simulink model "AEBWithSensorFusionMdlRef"  (R2020b)
settings: Solver=FixedStepAuto  StartTime=0.0  StopTime=34  FixedStep=0.1  RelTol=1e-3
undefined symbols (not defined in the file or in its folder): M, N, numCoasts, posSelector, speedController, Ts, v_set
libraries: drivinglib x2, pid_lib x1
settings Model: Creator=The MathWorks, Inc.  LastModifiedBy=chiar
settings SolverCC: MinimalZcImpactIntegration=on
settings DataIOCC: SaveOutput=off  SignalLogging=off  SaveTime=off  ReturnWorkspaceOutputs=off
settings OptimizationCC: DefaultParameterBehavior=Inlined  InlineInvariantSignals=on  PassReuseOutputArgsAs=Individual arguments  ZeroExternalMemoryAtStartup=off  ZeroInternalMemoryAtStartup=off  OptimizeBlockOrder=speed  EfficientTunableParamExpr=on
settings DebuggingCC: ParameterTunabilityLossMsg=error  ArithmeticOperatorsInVariantConditions=warning
settings HardwareCC: ProdLongLongMode=on
settings ModelReferenceCC: PropagateVarSize=Only when enabling
settings SFSimCC: SimUseLocalCustomCode=off  MATLABDynamicMemAlloc=off  CustomCodeUndefinedFunction=UseInterfaceOnly  SimTargetLang=C++
settings RTWCC: Description=Embedded Coder  SystemTargetFile=ert.tlc  TemplateMakefile=ert_default_tmf  GenerateReport=on  RTWUseLocalCustomCode=off  BuildConfiguration=Faster Runs  IncludeHyperlinkInReport=on  LaunchReport=on  TargetLang=C++  GenerateTraceInfo=on  GenerateTraceReport=on  GenerateTraceReportSl=on  GenerateTraceReportSf=on  GenerateTraceReportEml=on  GenerateCodeMetricsReport=on
settings CodeAppCC: ForceParamTrailComments=on  IgnoreCustomStorageClasses=off  MaxIdLength=63  OperatorAnnotations=on  SimulinkDataObjDesc=on  SFDataObjDesc=on  CustomSymbolStrFcn=$N$M$F  InsertBlockDesc=on
settings ERTTargetCC: TargetLangStandard=C++03 (ISO)  GenerateSampleERTMain=on  CombineSignalStateStructs=on  SuppressErrorStatus=on  CodeInterfacePackaging=C++ class  InlinedParameterPlacement=NonHierarchical  RootIOFormat=Structure reference  RTWCAPISignals=on  ERTCustomFileTemplate=example_file_process.tlc

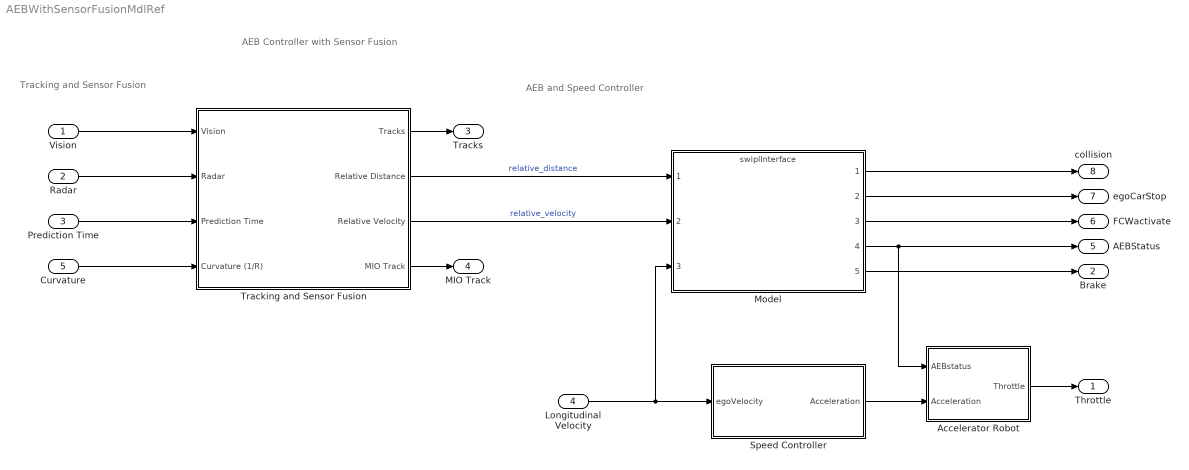
== system AEBWithSensorFusionMdlRef ==
  note: AEB and Speed Controller
  note: Tracking and Sensor Fusion
  note: AEB Controller with Sensor Fusion
  Vision : Inport  OutDataTypeStr=Bus: BusVision  PortDimensions=[1 1]  SampleTime=[0.10000000000000001,0]  BusOutputAsStruct=on
  Radar : Inport  Port=2  OutDataTypeStr=Bus: BusRadar  PortDimensions=[1 1]  SampleTime=[0.10000000000000001,0]  BusOutputAsStruct=on
  Prediction Time : Inport  Port=3  OutDataTypeStr=double  PortDimensions=[1 1]  SampleTime=[0.10000000000000001,0]  BusOutputAsStruct=on
  Longitudinal Velocity : Inport  Port=4  OutDataTypeStr=double  PortDimensions=1  SampleTime=[0.10000000000000001,0]
  Curvature : Inport  Port=5  OutDataTypeStr=double  PortDimensions=[1 1]  SampleTime=[0.10000000000000001,0]  BusOutputAsStruct=on
  Accelerator Robot : Subsystem
  Model : ModelReference  ModelNameDialog=swiplInterface.slx  SimulationMode=Normal  ModelReferenceVersion=1.2
  Speed Controller : Subsystem
  Tracking and Sensor Fusion : Subsystem  TreatAsAtomicUnit=on
      settings: RTWFileNameOpts=Use function name
  "Throttle " : Outport  OutDataTypeStr=double  PortDimensions=1  SampleTime=[0.10000000000000001,0]  VectorParamsAs1DForOutWhenUnconnected=off
  Brake : Outport  Port=2  OutDataTypeStr=double  PortDimensions=1  SampleTime=[0.10000000000000001,0]  VectorParamsAs1DForOutWhenUnconnected=off
  Tracks : Outport  Port=3  OutDataTypeStr=Bus:BusMultiObjectTracker1  PortDimensions=[1 1]  SampleTime=[0.10000000000000001,0]  VectorParamsAs1DForOutWhenUnconnected=off  BusOutputAsStruct=on
  MIO Track : Outport  Port=4  OutDataTypeStr=double  PortDimensions=1  SampleTime=[0.10000000000000001,0]  VectorParamsAs1DForOutWhenUnconnected=off
  AEBStatus : Outport  Port=5  OutDataTypeStr=uint8  PortDimensions=1  SampleTime=[0.10000000000000001,0]  VectorParamsAs1DForOutWhenUnconnected=off
  FCWactivate : Outport  Port=6  OutDataTypeStr=uint8  PortDimensions=1  SampleTime=[0.10000000000000001,0]  VectorParamsAs1DForOutWhenUnconnected=off
  egoCarStop : Outport  Port=7  PortDimensions=1  SampleTime=[0.10000000000000001,0]  VectorParamsAs1DForOutWhenUnconnected=off
  collision : Outport  Port=8  PortDimensions=1  SampleTime=[0.10000000000000001,0]  VectorParamsAs1DForOutWhenUnconnected=off
  wires:
  Tracking and Sensor Fusion/1(Tracks) -> Tracks/1
  Vision/1 -> Tracking and Sensor Fusion/1(Vision)
  Radar/1 -> Tracking and Sensor Fusion/2(Radar)
  Prediction Time/1 -> Tracking and Sensor Fusion/3(Prediction Time)
  Curvature/1 -> Tracking and Sensor Fusion/4(Curvature (1/R))
  Tracking and Sensor Fusion/4(MIO Track) -> MIO Track/1
  Longitudinal Velocity/1 -> Model/3, Speed Controller/1(egoVelocity)
  Tracking and Sensor Fusion/2(Relative Distance) -> Model/1  "relative_distance"
  Model/4 -> Accelerator Robot/1(AEBstatus), AEBStatus/1
  Tracking and Sensor Fusion/3(Relative Velocity) -> Model/2  "relative_velocity"
  Model/2 -> egoCarStop/1
  Model/1 -> collision/1
  Model/3 -> FCWactivate/1
  Model/5 -> Brake/1
  Speed Controller/1(Acceleration) -> Accelerator Robot/2(Acceleration)
  Accelerator Robot/1(Throttle) -> "Throttle "/1

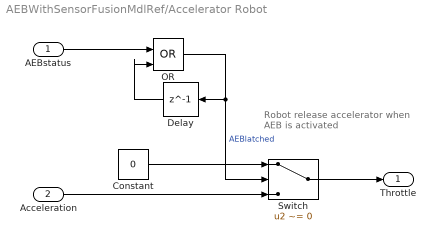
== system AEBWithSensorFusionMdlRef/Accelerator Robot ==
  note: Robot release accelerator when AEB is activated
  AEBstatus : Inport
  Acceleration : Inport  Port=2
  Constant : Constant  Value=0
  Delay : Delay  DelayLength=1
  OR : Logic  Operator=OR  IconShape=distinctive  AllPortsSameDT=off  OutDataTypeStr=boolean
  Switch : Switch  Criteria=u2 ~= 0
  Throttle : Outport  VectorParamsAs1DForOutWhenUnconnected=off
  wires:
  OR/1 -> Delay/1, Switch/2  "AEBlatched"
  Delay/1 -> OR/2
  Switch/1 -> Throttle/1
  AEBstatus/1 -> OR/1
  Constant/1 -> Switch/1
  Acceleration/1 -> Switch/3

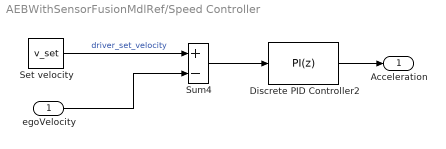
== system AEBWithSensorFusionMdlRef/Speed Controller ==
  egoVelocity : Inport
  Discrete PID Controller2 : pid_lib/PID Controller  Controller=PI  Form=Parallel  TimeDomain=Discrete-time  UseExternalTs=off  SampleTime=-1  IntegratorMethod=Forward Euler  FilterMethod=Forward Euler  ControllerParametersSource=internal  P=speedController.Kp  I=speedController.Ki  D=speedController.Kd  UseFilter=on  N=speedController.FilterCoeff  TunerSelectOption=Transfer Function Based (PID Tuner App)  InitialConditionSource=internal  InitialConditionForIntegrator=0  InitialConditionForFilter=0  DifferentiatorICPrevScaledInput=0  ExternalReset=none  TrackingMode=off  Kt=1  LimitOutput=on  SatLimitsSource=internal  UpperSaturationLimit=speedController.Amax  LowerSaturationLimit=speedController.Amin  LinearizeAsGain=off  AntiWindupMode=clamping  Kb=1  POutMin=[]  POutMax=[]  IOutMin=[]  IOutMax=[]  DOutMin=[]  DOutMax=[]  NOutMin=[]  NOutMax=[]  SumOutMin=[]  SumOutMax=[]  SaturationOutMin=[]  SaturationOutMax=[]  PParamMin=[]  PParamMax=[]  IParamMin=[]  IParamMax=[]  DParamMin=[]  DParamMax=[]  NParamMin=[]  NParamMax=[]  KbParamMin=[]  KbParamMax=[]  KtParamMin=[]  KtParamMax=[]  KbOutMin=[]  KbOutMax=[]  KtOutMin=[]  KtOutMax=[]  IntegratorOutMin=[]  IntegratorOutMax=[]  FilterOutMin=[]  FilterOutMax=[]  SumI1OutMin=[]  SumI1OutMax=[]  SumI2OutMin=[]  SumI2OutMax=[]  SumI3OutMin=[]  SumI3OutMax=[]  SumI4OutMin=[]  SumI4OutMax=[]  SumDOutMin=[]  SumDOutMax=[]  DifferentiatorOutMin=[]  DifferentiatorOutMax=[]  FilterDiffOutCoefMin=[]  FilterDiffOutCoefMax=[]  ReciprocalOutMin=[]  ReciprocalOutMax=[]  SumDenOutMin=[]  SumDenOutMax=[]  SumNumOutMin=[]  SumNumOutMax=[]  DivideOutMin=[]  DivideOutMax=[]  UdiffTsProdOutMin=[]  UdiffTsProdOutMax=[]  NTsProdOutMin=[]  NTsProdOutMax=[]  UintegralTsProdOutMin=[]  UintegralTsProdOutMax=[]  UngainTsProdOutMin=[]  UngainTsProdOutMax=[]  IntegratorContinuousStateAttributes=''  IntegratorStateMustResolveToSignalObject=off  IntegratorRTWStateStorageClass=Auto  FilterContinuousStateAttributes=''  FilterStateMustResolveToSignalObject=off  FilterRTWStateStorageClass=Auto  ParallelPVariant=InternalParameters  IdealPVariant=Disabled  IVariant=InternalParameters  DVariant=Disabled  IntegratorVariant=Discrete  SatVariant=Enabled  AWVariant=DiscClampingParallel  PCopyVariant=Disabled  TRVariant=Disabled  FdbkBlocksVariant=Forward  IdealPFdbkVariant=Disabled  SatFdbkVariant=Disabled  DerivativeFilterVariant=Disabled  NVariant=Disabled  NCopyVariant=Disabled_SignalSpec  FilterICVariant=Disabled  IntegratorICVariant=InternalICs  ExternalResetVariant=Disabled  TRSumVariant=Passthrough  SumFdbkVariant=Disabled  SumVariant=Sum_PI  TsampFilterVariant=InternalTs  TsampNgainVariant=Passthrough  TsampIntegralVariant=Passthrough  ExternalSaturationOutDataTypeStr=Inherit: Same as second input
  Set velocity : Constant  Value=v_set  SampleTime=Ts
  Sum4 : Sum  Inputs=+-
  Acceleration : Outport  VectorParamsAs1DForOutWhenUnconnected=off
  wires:
  Set velocity/1 -> Sum4/1  "driver_set_velocity"
  egoVelocity/1 -> Sum4/2
  Discrete PID Controller2/1 -> Acceleration/1
  Sum4/1 -> Discrete PID Controller2/1

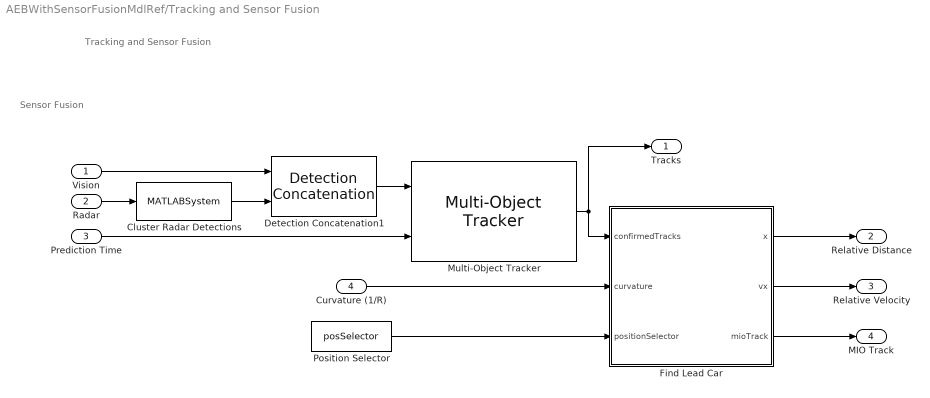
== system AEBWithSensorFusionMdlRef/Tracking and Sensor Fusion ==
  note: Sensor Fusion
  note: Tracking and Sensor Fusion
  Vision : Inport  OutDataTypeStr=Bus: BusVision  PortDimensions=[1 1]  SampleTime=[0.10000000000000001,0]  BusOutputAsStruct=on
  Radar : Inport  Port=2  OutDataTypeStr=Bus: BusRadar  PortDimensions=[1 1]  SampleTime=[0.10000000000000001,0]  BusOutputAsStruct=on
  Prediction Time : Inport  Port=3  OutDataTypeStr=double  PortDimensions=[1 1]  SampleTime=[0.10000000000000001,0]  BusOutputAsStruct=on
  Curvature (1/R) : Inport  Port=4  OutDataTypeStr=double  PortDimensions=[1 1]  SampleTime=[0.10000000000000001,0]  BusOutputAsStruct=on
  Cluster Radar Detections : MATLABSystem  System=helperClusterDetections  ClusterSize=clusterSize  BusNameSource=Auto  BusName=BusClusterDetections  SimulateUsing=Interpreted execution
      mask Type: helperClusterDetections
      mask Display:
      | disp(['Detection' char(10) 'Clustering']);
      | port_label('input',1,'In');
      | port_label('output',1,'Out');
  Detection Concatenation1 : drivinglib/Detection Concatenation  NumInputs=2  BusNameSource=Auto  BusName=BusDetectionConcatenation1  SimulateUsing=Interpreted execution
      settings: SourceProductName=Automated Driving Toolbox
  Find Lead Car : MATLAB Function  TreatAsAtomicUnit=on
  Multi-Object Tracker : drivinglib/Multi-Object Tracker  TrackerIndex=uint32( 0 )  FilterInitializationFcn=initcvekf  AssignmentThreshold=assigThresh  ConfirmationThreshold=[M,N]  DeletionThreshold=[numCoasts,numCoasts]  MaxNumTracks=numTracks  MaxNumSensors=numSensors  StateParams=struct  TimeInputSource=Input port  HasCostMatrixInput=off  HasDetectableTrackIDsInput=off  BusNameSource=Property  BusName=BusMultiObjectTracker1  TentativeTracksOutputPort=off  AllTracksOutputPort=off  SimulateUsing=Interpreted execution
      settings: SourceProductName=Automated Driving Toolbox
  Position Selector : Constant  Value=posSelector
  Tracks : Outport  OutDataTypeStr=Bus:BusMultiObjectTracker1  PortDimensions=[1 1]  SampleTime=[0.10000000000000001,0]  VectorParamsAs1DForOutWhenUnconnected=off  BusOutputAsStruct=on
  Relative Distance : Outport  Port=2  VectorParamsAs1DForOutWhenUnconnected=off
  Relative Velocity : Outport  Port=3  VectorParamsAs1DForOutWhenUnconnected=off
  MIO Track : Outport  Port=4  VectorParamsAs1DForOutWhenUnconnected=off
  wires:
  Find Lead Car/3(mioTrack) -> MIO Track/1
  Cluster Radar Detections/1 -> Detection Concatenation1/2
  Vision/1 -> Detection Concatenation1/1
  Prediction Time/1 -> Multi-Object Tracker/2
  Find Lead Car/2(vx) -> Relative Velocity/1
  Radar/1 -> Cluster Radar Detections/1
  Curvature (1/R)/1 -> Find Lead Car/2(curvature)
  Multi-Object Tracker/1 -> Find Lead Car/1(confirmedTracks), Tracks/1
  Detection Concatenation1/1 -> Multi-Object Tracker/1
  Find Lead Car/1(x) -> Relative Distance/1
  Position Selector/1 -> Find Lead Car/3(positionSelector)

== matlab function AEBWithSensorFusionMdlRef/Tracking and Sensor Fusion/Find Lead Car ==
  data: confirmedTracks input; x output double size=[1 1]; vx output size=[1 1]; curvature input; mioTrack output; positionSelector input
function [x,vx,mioTrack] = findLeadCar(confirmedTracks, curvature, positionSelector)
% This function finds the lead car: a car in front of the ego car that
% satisfies all the criteria below:
% * Within the ego car's lane.
% * In front of the ego car.
% * Closest to the ego car.

% Important notes:
% 1. If you change state definition, change the following:
%       State = [x;vx;y;vy;z;vz] (3D constant velocity)
numStates = 6;

% 2. The lane is defined using a parabolic model, where y=ax^2+bx+c. a is
%    equal to half the road curvature, b=0, and c is the offset of the lane
%    boundaries relative to the ego car. Overall lane width is assumed to
%    be 3.6m, typical highway lane width.
laneWidth = 3.6;

% 3. The ego car is assumed to be traveling in the middle of its lane, with
%    1.8m on each side of it. So, c=+1.8m for the left lane boundary and
%    -1.8m for the right lane boundary.
halfLaneWidth = laneWidth/2;

% Initialize outputs and parameters
maxX = cast(1000, 'like', confirmedTracks.Tracks(1).State);  % Far enough forward so that no track is expected to exceed this distance
trackID = 0;

for i = 1:confirmedTracks.NumTracks
    position = positionSelector * confirmedTracks.Tracks(i).State;
    x = position(1); % Longitudinal position of the track relative to ego
    y = position(2); % Lateral position of the track relative to ego
    
    if x < maxX && x > 0 % No point checking otherwise
        yleftLane  = polyval([curvature/2, 0,  halfLaneWidth],x); % Half a lane to the left
        yrightLane = polyval([curvature/2, 0, -halfLaneWidth],x); % Half a lane to the right
        
        % Find a new lead car
        if (yrightLane <= y) && (y <= yleftLane)
            maxX = x;
            trackID = i;
        end
    end
end

if trackID>0
    mioState = confirmedTracks.Tracks(trackID).State;
else
    mioState = inf(numStates,1,'like',confirmedTracks.Tracks(1).State);
end

% Output:
x = mioState(1);    % Longitudinal position of the lead car
vx = mioState(2);   % Longitudinal velocity of the lead car
mioTrack = trackID; % Index of the most important track
